simulink model "sim_model"  (R2017a)
settings: Solver=ode23s  StartTime=0.0  StopTime=8  RelTol=1e-7  AbsTol=1e-9
values from neighbouring files (symbols this model uses):
  A = [0 1;0 0]    [ex01_linear_state_and_input_constraints.m]    (also in ex02_multiregion.m = kron(eye(2),[0 1;0 0]); ex02_polyhedral.m = kron(eye(2),[0 1;0 0]))
  B = [0;1]    [ex01_linear_state_and_input_constraints.m]    (also in ex02_multiregion.m = kron(eye(2),[0;1]); ex02_polyhedral.m = kron(eye(2),[0;1]))
  F = [-w^2 -2*z*w]    [ex01_linear_state_and_input_constraints.m]    (also in ex02_multiregion.m = kron(eye(2),[-w^2 -2*xi*w]); ex02_polyhedral.m = kron(eye(2),[-w^2 -2*xi*w]))
  G = w^2    (= 100)    [ex01_linear_state_and_input_constraints.m]    (also in ex02_multiregion.m = kron(eye(2),w^2); ex02_polyhedral.m = kron(eye(2),w^2))
  x0 = [0 0]'    [ex01_linear_state_and_input_constraints.m]    (also in ex02_multiregion.m = [-.7 0 -.7 0]'; ex02_polyhedral.m = [-.7 0 -.7 0]')
libraries: ERG_lib x1
settings Model: Creator=Admin  LastModifiedBy=Admin

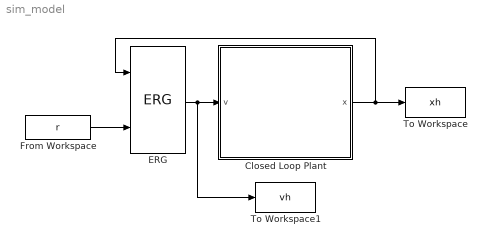
== system sim_model ==
  Closed Loop Plant : Subsystem
  ERG : ERG_lib/ERG  erg_param=erg  kappa_param=1000
  From Workspace : FromWorkspace  VariableName=r  SampleTime=0
  To Workspace : ToWorkspace  VariableName=xh  SaveFormat=Timeseries  SampleTime=-1
  To Workspace1 : ToWorkspace  VariableName=vh  SaveFormat=Timeseries  SampleTime=-1
  wires:
  Closed Loop Plant/1(x) -> ERG/1, To Workspace/1
  From Workspace/1 -> ERG/2
  ERG/1 -> To Workspace1/1, Closed Loop Plant/1(v)

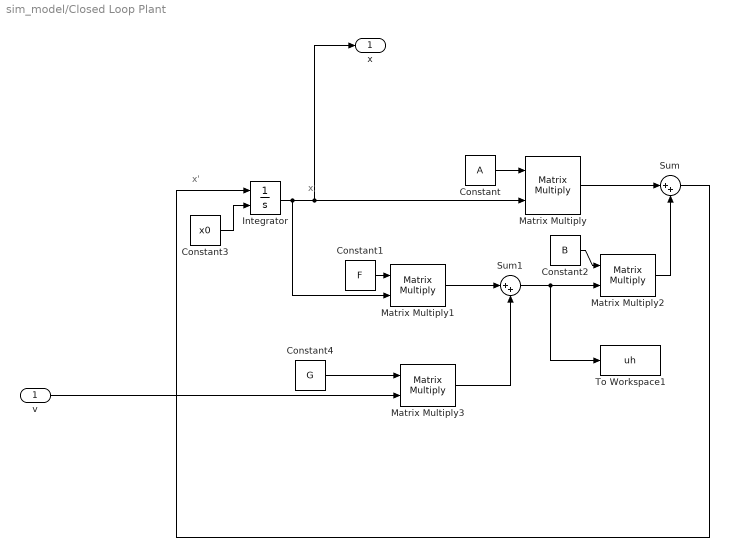
== system sim_model/Closed Loop Plant ==
  note: x'
  note: x
  v : Inport
  Constant : Constant  Value=A
  Constant1 : Constant  Value=F  VectorParams1D=off
  Constant2 : Constant  Value=B  VectorParams1D=off
  Constant3 : Constant  Value=x0  VectorParams1D=off
  Constant4 : Constant  Value=G  VectorParams1D=off
  Integrator : Integrator  InitialConditionSource=external  InitialCondition=x0
  Matrix Multiply{,1..3} (4 alike) : Product  Multiplication=Matrix(*)
  Sum : Sum  Inputs=|++
  Sum1 : Sum  Inputs=|++
  To Workspace1 : ToWorkspace  VariableName=uh  SaveFormat=Timeseries  SampleTime=-1
      settings: Save2DSignal=2-D array (concatenate along first dimension)
  x : Outport
  wires:
  Matrix Multiply1/1 -> Sum1/1
  Matrix Multiply3/1 -> Sum1/2
  Sum1/1 -> Matrix Multiply2/2, To Workspace1/1
  v/1 -> Matrix Multiply3/2
  Constant4/1 -> Matrix Multiply3/1
  Constant1/1 -> Matrix Multiply1/1
  Integrator/1 -> Matrix Multiply1/2, x/1, Matrix Multiply/2
  Sum/1 -> Integrator/1
  Matrix Multiply2/1 -> Sum/2
  Constant3/1 -> Integrator/2
  Matrix Multiply/1 -> Sum/1
  Constant/1 -> Matrix Multiply/1
  Constant2/1 -> Matrix Multiply2/1
